simulink model "DSBFC_SIM"  (R2018a)
settings: Solver=VariableStepAuto  StartTime=0.0  StopTime=10.0  RelTol=1e-3
libraries: dsparch4 x1
settings Model: Creator=vnrvjiet  LastModifiedBy=vnrvjiet

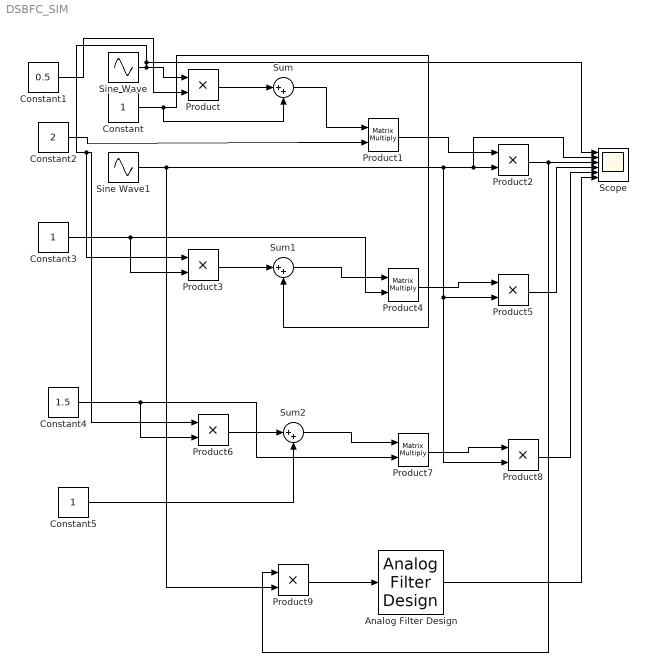
== system DSBFC_SIM ==
  Analog Filter Design : dsparch4/Analog Filter Design  method=Butterworth  filttype=Lowpass  N=8  Wlo=2*pi*10  Whi=80  Rp=2  Rs=40
  Constant : Constant
  Constant1 : Constant  Value=0.5
  Constant2 : Constant  Value=2
  Constant3 : Constant
  Constant4 : Constant  Value=1.5
  Constant5 : Constant
  Product{,2..3,5..6,8..9} (7 alike) : Product
  Product1 : Product  Multiplication=Matrix(*)
  Product4 : Product  Multiplication=Matrix(*)
  Product7 : Product  Multiplication=Matrix(*)
  Scope : Scope  NumInputPorts=6
  Sine Wave : Sin  Frequency=2*pi*10  SampleTime=1/1000
  Sine Wave1 : Sin  Frequency=2*pi*200  SampleTime=1/1000
  Sum : Sum  Inputs=|++
  Sum1 : Sum  Inputs=|++
  Sum2 : Sum  Inputs=|++
  wires:
  Sine Wave/1 -> Product6/1, Product3/1, Scope/1, Product/1
  Constant/1 -> Sum1/2, Sum/2
  Product/1 -> Sum/1
  Sum/1 -> Product1/1
  Product1/1 -> Product2/1
  Sine Wave1/1 -> Product8/2, Product5/2, Product2/2, Scope/2, Product9/2
  Product2/1 -> Product9/1, Scope/3
  Constant1/1 -> Product/2
  Constant2/1 -> Product1/2
  Constant3/1 -> Product4/2, Product3/2
  Product3/1 -> Sum1/1
  Sum1/1 -> Product4/1
  Product4/1 -> Product5/1
  Product5/1 -> Scope/4
  Product7/1 -> Product8/1
  Sum2/1 -> Product7/1
  Product6/1 -> Sum2/1
  Constant4/1 -> Product7/2, Product6/2
  Constant5/1 -> Sum2/2
  Product8/1 -> Scope/5
  Product9/1 -> Analog Filter Design/1
  Analog Filter Design/1 -> Scope/6
